simulink model "uav_simple_flight_model9"  (R2024b)
settings: Solver=VariableStepAuto  StartTime=0.0  StopTime=30  RelTol=1e-3
undefined symbols (not defined in the file or in its folder): gray, Sim3dSensor
libraries: simulink x3, robotcorelib x1, visionsinks x1, sim3dautolib x1, sim3dcameralib x1, sim3dlib x1, uavsim3dlib x1, visionanalysis x1, uavutilslib x1
settings Model: Creator=Cihan_Sevgili  LastModifiedBy=Cihan_Sevgili
settings RTWCC: GPUComputeCapability=3.5

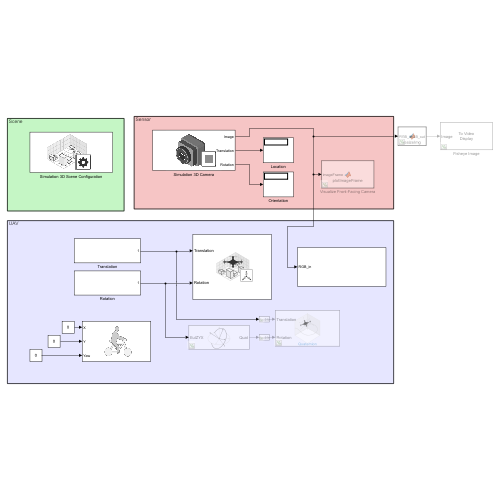
[thumbnail: Simulink's stored preview of the top-level diagram]
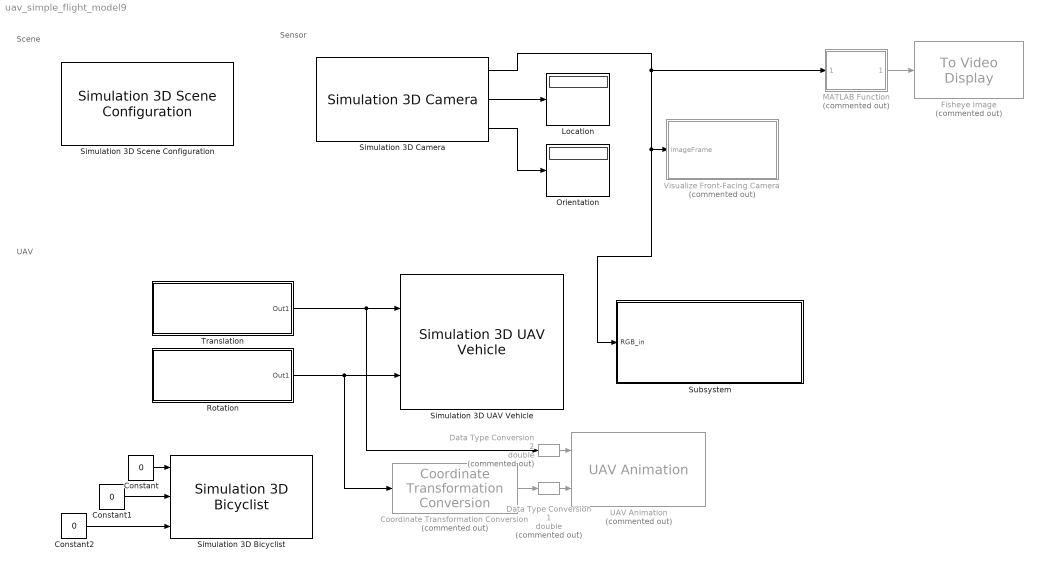
== system uav_simple_flight_model9 ==
  note: UAV
  note: Sensor
  note: Scene
  Constant : Constant  Value=0
  Constant1 : Constant  Value=0
  Constant2 : Constant  Value=0
  Coordinate Transformation Conversion : robotcorelib/Coordinate Transformation Conversion  Commented=on  InputRepresentation=Euler Angles  InputEulerSequence=ZYX  ShowTrVecInputPort=on  OutputRepresentation=Quaternion  OutputEulerSequence=ZYX  ShowTrVecOutputPort=on  SimulateUsing=Code generation
  Data Type Conversion1 : DataTypeConversion  Commented=on  OutDataTypeStr=double  SaturateOnIntegerOverflow=off  RndMeth=Floor
  Data Type Conversion2 : DataTypeConversion  Commented=on  OutDataTypeStr=double  SaturateOnIntegerOverflow=off  RndMeth=Floor
  Fisheye Image : visionsinks/To Video Display  Commented=on  windowSizeMode=Normal  openAtMdlStart=on  fullScreen=off  videoWindowX=693  videoWindowY=238  saveWindowSize=off  videoWindowWidth=691  videoWindowHeight=692  inputColorFormat=RGB  inputType=Obsolete  imagePorts=One multidimensional signal  OutputDevice=On-screen video monitor  dataOrg=Column-major  isWindowOpen=off
  Location : Display
  MATLAB Function : MATLAB Function  Commented=on  TreatAsAtomicUnit=on
  Orientation : Display
  Rotation : Subsystem
  Simulation 3D Bicyclist : sim3dautolib/Simulation 3D Bicyclist  Priority=-1  Scale=[1, 1, 1]  InitialPos=[0, 0, 0]  InitialRot=[0, 0, 0]  ActorName=SimulinkBicyclist1  SampleTime=-1  ActorType=SimulinkBicyclist  ActorTag=SimulinkBicyclist1  ID=1  aMode=3  CoordinateScheme=ISO  TransformOutportEnabled=off
      settings: LibrarySourceBlock=drivingsim3d/Simulation 3D Bicyclist
  Simulation 3D Camera : sim3dcameralib/Simulation 3D Camera  Priority=1  sensorTag=Sim3dSensor�  sensorId=1  sensorName=Sim3dSensor�  vehTagList={'Scene Origin';'SimulinkVehicle1'}  vehTag=SimulinkVehicle1  mountLoc=Origin  offsetFlag=on  tmountOffset=[0.1, 0, 0]  extTmount=off  rmountOffset=[0, 0, 0]  extRmount=off  FocalLength=[1109, 1109]  OpticalCenter=[320, 180]%[640, 360]  ImageSize=[360, 640]%[720, 1280]  RadialDistortion=[0, 0]  TangentialDistortion=[0, 0]  SensorSkew=0  DepthOutportEnabled=off  SemanticOutportEnabled=off  TransformOutportEnabled=on  SampleTime=-1  mountPoint=[0.1 0 0]  mountOrientation=[0 0 0]  aMode=4  ID=1
      settings: LibrarySourceBlock=uavsim3dlib/Simulation 3D Camera
  Simulation 3D Scene Configuration : sim3dlib/Simulation 3D Scene Configuration  Priority=0  ProjectFormat=Default Scenes  SceneDesc=US city block  ProjectName=C:\Program Files\MATLAB\R2024b\toolbox\shared\sim3d_projects\automotive_project_windows\UE\WindowsNoEditor\VehicleSimulation.exe  ScenePath=/Game/Maps/USCityBlock  EnableOpenDRIVE=off  vehTagList={'Custom';'Scene Origin';'SimulinkVehicle1'}  vehTag=Scene Origin  FreeCameraInitialTranslation=[0, 0, 0]  FreeCameraDefaultInitialTranslation=[-6, 0, 2]  FreeCameraInitialRotation=[0, 0, 0]  FreeCameraDefaultInitialRotation=[0, -15, 0]  OpVisEn=off  Ts=1/4  EnableWindow=off  EnableRemoteAccess=off  EnableWeather=off  SunAzimuth=90  SunAltitude=40.0  EnableGeospatialSun=off  Latitude=0  Longitude=0  Date=2023-01-01  Time=10:30:00  GeoTimeZone=-5.0  SunDaylightSaving=off  wind=1  clouds=10  EnableVolumetricClouds=off  CloudCoverage=0  CloudAltitude=6  fog=0  rain=0  RaindropsEffect=off  SnowDensity=0  EnableGeospatial=off  UseTrueOrigin=off  OriginHeight=200  OriginLatitude=40.744652  OriginLongitude=-73.988864  MapStyle=Aerial  AdditionalAssetIDs=[]  UseAdvancedSunSky=off  SolarTime=11  TimeZone=-5  Day=21  Month=9  Year=2022  UseDaylightSavingTime=on  DSTStartDay=10  DSTStartMonth=3  DSTEndDay=3  DSTEndMonth=11  DSTSwitchHour=2  sensorTag=MainCamera1  sensorId=1  sensorName=MainCamera1  mountLoc=Origin  offsetFlag=off  tmountOffset=[0, 0, 0]  rmountOffset=[0, 0, 0]  HorizontalResolution=1280  VerticalResolution=720  HorizontalFOV=60  mountPoint=[0 0 0]  mountOrientation=[0 0 0]  aMode=4  ID=1  GeoTrigger=Inactive
      settings: LibrarySourceBlock=uavsim3dlib/Simulation 3D Scene Configuration
  Simulation 3D UAV Vehicle : uavsim3dlib/Simulation 3D UAV Vehicle  Mesh=Quadrotor  MeshPath=/MathWorksUAVContent/UAVs/HexaRotorUAV/HexaRotor.HexaRotor  Color=Black  ActorName=SimulinkVehicle1  UseGlobalFrame=off  InitialTranslation=[0 5 1.5]  InitialRotation=[0 0 0]  InitialTranslationGlobal=[0 0 0]  InitialGeoOrigin=[0 0 0]  InitialRotationGlobal=[0 0 0]  SampleTime=-1  ActorType=SimulinkVehicle  ID=1  aMode=4  ActorTag=SimulinkVehicle1
  Subsystem : Subsystem
  Translation : Subsystem
  UAV Animation : uavutilslib/UAV Animation  Commented=on  NumUAV=1  DynamicUAVConfig=off  UAVType=Multirotor  UAVSize=1  UAVColor=[1 0 0]  UAVTrajectoryAlpha=1  InertialZDirection=Down  RotationFormat=Quaternion  DrawMarkers=off  SampleTime=-1
  Visualize Front-Facing Camera : MATLAB Function  Commented=on  TreatAsAtomicUnit=on
  wires:
  Data Type Conversion1/1 -> UAV Animation/2
  Simulation 3D Camera/3 -> Orientation/1
  Translation/1(Out1) -> Data Type Conversion2/1, Simulation 3D UAV Vehicle/1
  Data Type Conversion2/1 -> UAV Animation/1
  Simulation 3D Camera/2 -> Location/1
  Simulation 3D Camera/1 -> Subsystem/1(RGB_in), Visualize Front-Facing Camera/1(imageFrame), MATLAB Function/1(RGB_in)
  Rotation/1(Out1) -> Simulation 3D UAV Vehicle/2, Coordinate Transformation Conversion/1
  Constant/1 -> Simulation 3D Bicyclist/1
  Constant2/1 -> Simulation 3D Bicyclist/3
  Constant1/1 -> Simulation 3D Bicyclist/2
  Coordinate Transformation Conversion/1 -> Data Type Conversion1/1
  MATLAB Function/1(RGB_out) -> Fisheye Image/1

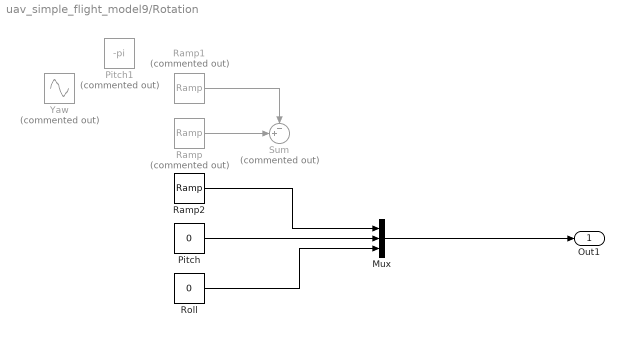
== system uav_simple_flight_model9/Rotation ==
  Mux : Mux  Inputs=3
  Pitch : Constant  Value=0
  Pitch1 : Constant  Commented=on  Value=-pi
  Ramp : simulink/Sources/Ramp  Commented=on  slope=pi/45  start=0  InitialOutput=pi/6
  Ramp1 : simulink/Sources/Ramp  Commented=on  slope=2*pi/45  start=15  InitialOutput=0
  Ramp2 : simulink/Sources/Ramp  slope=-pi/45  start=0  InitialOutput=5*pi/6
  Roll : Constant  Value=0
  Sum : Sum  Commented=on  Inputs=-+|
  Yaw : Sin  Commented=on  Amplitude=-2  Frequency=1.5*(pi/(18*4))/2  Phase=-pi/2+pi/12  SampleTime=0
  Out1 : Outport
  wires:
  Pitch/1 -> Mux/2
  Roll/1 -> Mux/3
  Mux/1 -> Out1/1
  Ramp/1 -> Sum/2
  Ramp1/1 -> Sum/1
  Ramp2/1 -> Mux/1

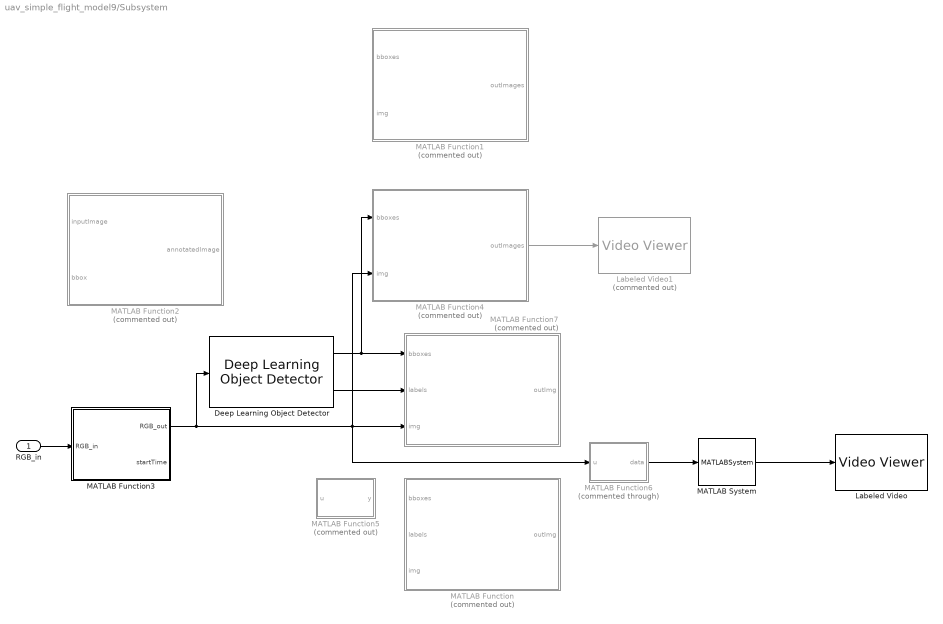
== system uav_simple_flight_model9/Subsystem ==
  RGB_in : Inport
  Deep Learning Object Detector : visionanalysis/Deep Learning Object Detector  Detector=Detector from MAT-file  DetectorFunction=untitled  DetectorFilePath=D:\ControlCode\Sandbox\MatlabBiker\reforgeddata\labeler224.mat  MaxDetections=500  Bboxes=on  Scores=off  UseROI=off  AutoResize=on  ROI=[1 1 100 100]  Threshold=0.75  NumStrongestRegions=2000  UseMinSize=off  MinSize=[1 1]  UseMaxSize=off  MaxSize=[50 50]  ForceInterpretedSim=off
  Labeled Video : VideoViewer  colormapValue=gray(256)  FigPos=[1 1030 1920 930]
  Labeled Video1 : VideoViewer  Commented=on  colormapValue=gray(256)  FigPos=[1 1078 918 790]
  MATLAB Function : MATLAB Function  Commented=on  TreatAsAtomicUnit=on
  MATLAB Function1 : MATLAB Function  Commented=on  TreatAsAtomicUnit=on
  MATLAB Function2 : MATLAB Function  Commented=on  TreatAsAtomicUnit=on
  MATLAB Function3 : MATLAB Function  TreatAsAtomicUnit=on
  MATLAB Function4 : MATLAB Function  Commented=on  TreatAsAtomicUnit=on
  MATLAB Function5 : MATLAB Function  Commented=on  TreatAsAtomicUnit=on
  MATLAB Function6 : MATLAB Function  Commented=through  TreatAsAtomicUnit=on
  MATLAB Function7 : MATLAB Function  Commented=on  TreatAsAtomicUnit=on
  MATLAB System : MATLABSystem  System=SaveImageToWorkspace  SimulateUsing=Interpreted execution
      mask Type: SaveImageToWorkspace
      mask Display:
      | disp('SaveImageToWorkspace');
      | port_label('input',1,'u');
      | port_label('output',1,'y');
  wires:
  RGB_in/1 -> MATLAB Function3/1(RGB_in)
  MATLAB Function3/1(RGB_out) -> MATLAB Function7/3(img), MATLAB Function6/1(u), MATLAB Function4/2(img), Deep Learning Object Detector/1
  Deep Learning Object Detector/1 -> MATLAB Function4/1(bboxes), MATLAB Function7/1(bboxes)
  MATLAB Function4/1(outImages) -> Labeled Video1/1
  Deep Learning Object Detector/2 -> MATLAB Function7/2(labels)
  MATLAB Function6/1(data) -> MATLAB System/1
  MATLAB System/1 -> Labeled Video/1

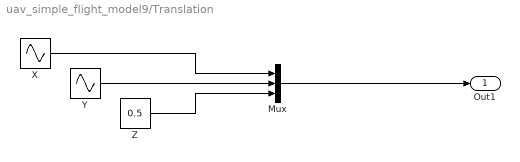
== system uav_simple_flight_model9/Translation ==
  Mux : Mux  Inputs=3
  X : Sin  Amplitude=3  Frequency=2*pi/90 %1.5*pi/(18*4)  Phase=pi/2+pi/6  SampleTime=0
  Y : Sin  Amplitude=3  Frequency=2*pi/90 %1.5*pi/(18 *4)  Phase=pi+pi/6  SampleTime=0
  Z : Constant  Value=0.5
  Out1 : Outport
  wires:
  Y/1 -> Mux/2
  Z/1 -> Mux/3
  X/1 -> Mux/1
  Mux/1 -> Out1/1

== matlab function uav_simple_flight_model9/Subsystem/MATLAB Function1 ==
  data: bboxes input; outImages output; img input
function outImages = AnnotateAndCropImage(bboxes, img)
    %#codegen
    
    % Input validation
    validateattributes(img, {'uint8'}, {'size',[416,416,3]});
    validateattributes(bboxes, {'single','double'}, {'size',[1,4]});
    
    % Define fixed sizes
    cropSize = [208, 208, 3];
    maxBoxes = 1; % Set to maximum number of boxes you expect
    
    % Pre-allocate output with fixed size
    outImages = zeros([cropSize, maxBoxes], 'uint8');
    
    % Ensure we don't exceed maxBoxes
    numBoxes = min(size(bboxes, 1), maxBoxes);
    
    for i = 1:numBoxes
        % Extract bbox coordinates
        x = max(1, round(bboxes(i, 1)));
        y = max(1, round(bboxes(i, 2)));
        width = round(bboxes(i, 3));
        height = round(bboxes(i, 4));
        
        % Ensure coordinates are within image bounds
        x2 = min(x + width - 1, size(img, 2));
        y2 = min(y + height - 1, size(img, 1));
        
        % Crop the region inside the bounding box
        croppedImg = img(y:y2, x:x2, :);
        
        % Resize cropped image to fixed size
        resizedCrop = imresize(croppedImg, cropSize(1:2));
        
        % Store in output array
        outImages(:, :, :, i) = resizedCrop;
    end
end

== matlab function uav_simple_flight_model9/Subsystem/MATLAB Function2 ==
  data: inputImage input; bbox input; annotatedImage output
function annotatedImage = cropBoundingBox(inputImage, bbox)
    %#codegen
    
    % Use coder.ignoreConst for runtime validation
    coder.inline('never');
    validateattributes(bbox, {'double','single'}, {'size',[1,4]});
    validateattributes(inputImage, {'uint8','single'}, {'size',[NaN,NaN,3]});
    
    % Define sizes
    cropSize = [416 416];
    targetSize = [208 208];
    
    % Calculate center crop position
    [imgHeight, imgWidth, ~] = size(inputImage);
    startX = floor((imgWidth - cropSize(2)) / 2) + 1;
    startY = floor((imgHeight - cropSize(1)) / 2) + 1;
    
    % Crop the image manually
    J = inputImage(startY:startY+cropSize(1)-1, startX:startX+cropSize(2)-1, :);
    
    % Adjust bounding box coordinates relative to crop window
    bbox_x = bbox(1) - startX + 1;
    bbox_y = bbox(2) - startY + 1;
    bbox_w = bbox(3);
    bbox_h = bbox(4);
    
    % Clip bbox to crop window bounds
    bbox_x = max(1, min(bbox_x, cropSize(2)));
    bbox_y = max(1, min(bbox_y, cropSize(1)));
    bbox_w = min(bbox_w, cropSize(2) - bbox_x + 1);
    bbox_h = min(bbox_h, cropSize(1) - bbox_y + 1);
    
    % Scale factors for resizing
    scale_x = targetSize(2) / cropSize(2);
    scale_y = targetSize(1) / cropSize(1);
    
    % Resize image using imresize
    J = imresize(J, targetSize);
    
    % Scale bounding box coordinates
    bbox_x = round(bbox_x * scale_x);
    bbox_y = round(bbox_y * scale_y);
    bbox_w = round(bbox_w * scale_x);
    bbox_h = round(bbox_h * scale_y);
    
    % Create output image
    annotatedImage = J;
    
    % Draw rectangle manually (fixed version)
    lineWidth = 2;
    redChannel = uint8(255);
    greenChannel = uint8(0);
    blueChannel = uint8(0);
    
    for i = max(1, bbox_y-lineWidth):min(targetSize(1), bbox_y+bbox_h+lineWidth)
        for j = max(1, bbox_x-lineWidth):min(targetSize(2), bbox_x+lineWidth)
            if j <= targetSize(2)
                annotatedImage(i,j,1) = redChannel;
                annotatedImage(i,j,2) = greenChannel;
                annotatedImage(i,j,3) = blueChannel;
            end
        end
        for j = max(1, bbox_x+bbox_w-lineWidth):min(targetSize(2), bbox_x+bbox_w+lineWidth)
            if j <= targetSize(2)
                annotatedImage(i,j,1) = redChannel;
                annotatedImage(i,j,2) = greenChannel;
                annotatedImage(i,j,3) = blueChannel;
            end
        end
    end
    
    for j = max(1, bbox_x-lineWidth):min(targetSize(2), bbox_x+bbox_w+lineWidth)
        for i = max(1, bbox_y-lineWidth):min(targetSize(1), bbox_y+lineWidth)
            if i <= targetSize(1)
                annotatedImage(i,j,1) = redChannel;
                annotatedImage(i,j,2) = greenChannel;
                annotatedImage(i,j,3) = blueChannel;
            end
        end
        for i = max(1, bbox_y+bbox_h-lineWidth):min(targetSize(1), bbox_y+bbox_h+lineWidth)
            if i <= targetSize(1)
                annotatedImage(i,j,1) = redChannel;
                annotatedImage(i,j,2) = greenChannel;
                annotatedImage(i,j,3) = blueChannel;
            end
        end
    end
end

== matlab function uav_simple_flight_model9/Visualize Front-Facing Camera ==
  data: imageFrame input
function plotImageFrame(imageFrame)
    grayFrame = rgb2gray(imageFrame);  % Convert to grayscale

    coder.extrinsic('ishandle','imshow');  % Use 'imshow' instead of 'image'
    
    persistent fig;
    
    if isempty(fig)
        fig = figure();
        ax = newplot(fig);
        title(ax, 'Front-facing camera');
    end

    if ~isempty(fig) && ishandle(fig)
        ax = newplot(fig);
        imshow(grayFrame, 'Parent', ax);  % Use 'imshow' and specify the parent axes
        axis(ax, 'off');  % Turn off the axes
    end
end

%%
%object detection using blob analysis

== matlab function uav_simple_flight_model9/Subsystem/MATLAB Function ==
  data: bboxes input; labels input; outImg output; img input
function outImg = AnnotateImage(bboxes, labels, img)
    % Annotate detections in the image. 

    if ~isempty(bboxes)
        for i = 1:numel(labels)
            img = insertObjectAnnotation(img, "rectangle", bboxes(i, :), char(labels(i)));
        end
    end

    outImg = img;

end

== matlab function uav_simple_flight_model9/Subsystem/MATLAB Function3 ==
  data: RGB_in input; RGB_out output; startTime output
function [RGB_out, startTime] = resizeImg(RGB_in)
    %RGB_out = imresize(RGB_in,[416,416]);
        RGB_out = RGB_in;

    currentTime = datetime;
    startTime = [currentTime.Year currentTime.Month currentTime.Day currentTime.Hour ...
        currentTime.Minute currentTime.Second];
end

== matlab function uav_simple_flight_model9/Subsystem/MATLAB Function6 ==
  data: u input; data output
function data = saveImageToWorkspace(u)
%#codegen
coder.extrinsic('assignin', 'sprintf');

persistent stepCounter
if isempty(stepCounter)
    stepCounter = int32(1);
end

if coder.target('MATLAB')
    stepStr = sprintf('%04d', stepCounter);
    varName = ['image_step_', stepStr];
    assignin('base', varName, uint8(u));
end

stepCounter = stepCounter + 1;
data = u;
end

== matlab function uav_simple_flight_model9/Subsystem/MATLAB Function4 ==
  data: bboxes input; outImages output; img input
function outImages = AnnotateAndCropImage(bboxes, img)
    %#codegen

    % Input validation with flexible sizes
    validateattributes(img, {'uint8'}, {'ndims', 3, 'size', [NaN, NaN, 3]}); % Flexible image size
    validateattributes(bboxes, {'single', 'double'}, {'ncols', 4}); % Allow any number of rows with 4 columns

    % Define fixed sizes for cropped output
    %cropSize = [416, 416, 3];
    cropSize = [720, 720, 3];
    maxBoxes = 1; % Adjust based on expected max number of bounding boxes

    % Pre-allocate output with fixed size
    outImages = zeros([cropSize, maxBoxes], 'uint8');

    % Ensure we don't exceed maxBoxes
    numBoxes = min(size(bboxes, 1), maxBoxes);

    for i = 1:numBoxes
        % Extract bounding box coordinates
        x = max(1, round(bboxes(i, 1)));
        y = max(1, round(bboxes(i, 2)));
        width = round(bboxes(i, 3));
        height = round(bboxes(i, 4));

        % Ensure coordinates are within image bounds
        x2 = min(x + width - 1, size(img, 2));
        y2 = min(y + height - 1, size(img, 1));

        % Crop the region inside the bounding box
        croppedImg = img(y:y2, x:x2, :);

        % Resize cropped image to fixed size
        resizedCrop = imresize(croppedImg, cropSize(1:2));

        % Store in output array
        outImages(:, :, :, i) = resizedCrop;
    end
end

== matlab function uav_simple_flight_model9/Subsystem/MATLAB Function5 ==
  data: u input; y output
function y = fcn(u)

y = u;

== matlab function uav_simple_flight_model9/Subsystem/MATLAB Function7 ==
  data: bboxes input; labels input; outImg output; img input
function outImg  = AnnotateImage(bboxes, labels, img)
    % Annotate detections in the image. 
    % Check if labels have at least three elements to perform swapping
    % disp(labels);
    % disp("numel")
    % disp(numel(labels))
    disp("labels")

 

    if ~isempty(bboxes)
        for i = 1:numel(labels)
            if (labels(i) == labeler224_labels.angle45_label)
                labels(i) = labeler224_labels.angle135_label;
            % elseif (labels(i)== "angle90_label")
            %     labels(i) = "angle45_label";
            elseif (labels(i) == labeler224_labels.angle90_label)
                labels(i) = labeler224_labels.angle45_label;                
            elseif (labels(i) == labeler224_labels.angle135_label)
                labels(i) = labeler224_labels.angle90_label;
            end
            disp(labels(i))
            img = insertObjectAnnotation(img, "rectangle", bboxes(i, :), char(labels(i)));
        end
    end

    outImg = img;

end

== matlab function uav_simple_flight_model9/MATLAB Function ==
  data: RGB_in input; RGB_out output
function RGB_out  = resizeImg(RGB_in)
    RGB_out = imresize(RGB_in,[416,416]);

end
